simulink model "week1_7"  (R2020b)
settings: Solver=VariableStepAuto  StartTime=0.0  StopTime=10.0  MaxStep=0.01  RelTol=1e-3
libraries: dspsrcs4 x1
settings Model: Creator=lalit  LastModifiedBy=lalit

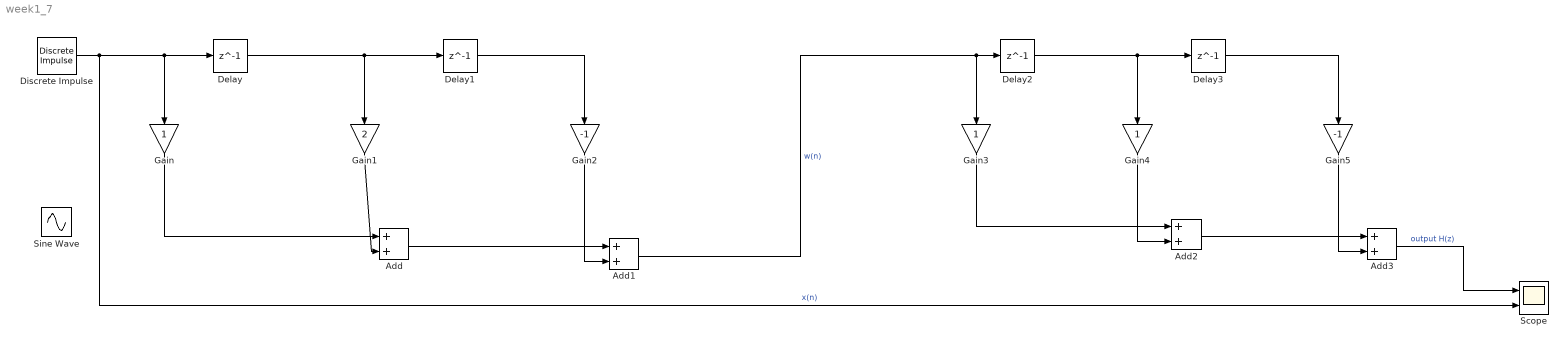
== system week1_7 ==
  Add{,1..3} (4 alike) : Sum
  Delay{,1..3} (4 alike) : Delay  DelayLength=1
  Discrete Impulse : dspsrcs4/Discrete  Impulse  Delay=0  SampleTime=1  FrameSample=1  OutputFrames=off  dataType=double  isSigned=on  wordLen=16  udDataType=sfix(16)  fracBitsMode=Best precision  numFracBits=15  OutDataTypeStr=double  LastOutDataTypeStr=double
  Gain : Gain
  Gain1 : Gain  Gain=2
  Gain2 : Gain  Gain=-1
  Gain3 : Gain
  Gain4 : Gain
  Gain5 : Gain  Gain=-1
  Scope : Scope  NumInputPorts=2
  Sine Wave : Sin  Amplitude=5  Frequency=10  SampleTime=0
  wires:
  Discrete Impulse/1 -> Scope/2, Gain/1, Delay/1  "x(n)"
  Delay/1 -> Gain1/1, Delay1/1
  Delay2/1 -> Gain4/1, Delay3/1
  Delay1/1 -> Gain2/1
  Delay3/1 -> Gain5/1
  Gain/1 -> Add/1
  Gain1/1 -> Add/2
  Add/1 -> Add1/1
  Gain2/1 -> Add1/2
  Add1/1 -> Gain3/1, Delay2/1  "w(n)"
  Gain3/1 -> Add2/1
  Gain4/1 -> Add2/2
  Add2/1 -> Add3/1
  Gain5/1 -> Add3/2
  Add3/1 -> Scope/1  "output H(z)"
